simulink model "CORREC_OTLADKA"  (R2023a)
settings: Solver=VariableStepAuto  StartTime=0.0  StopTime=0.1  RelTol=1e-3
settings Model: Creator=ycheb  LastModifiedBy=ycheb

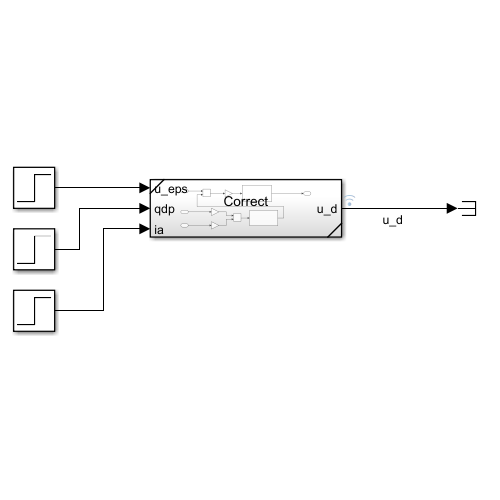
[thumbnail: Simulink's stored preview of the top-level diagram]
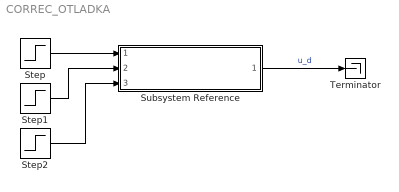
== system CORREC_OTLADKA ==
  Step : Step  Time=0  SampleTime=0
  Step1 : Step  Time=0  SampleTime=0
  Step2 : Step  Time=0  SampleTime=0
  Subsystem Reference : Subsystem  ReferencedSubsystem=Correct
  Terminator : Terminator
  wires:
  Step/1 -> Subsystem Reference/1
  Subsystem Reference/1 -> Terminator/1  "u_d"
  Step2/1 -> Subsystem Reference/3
  Step1/1 -> Subsystem Reference/2
